simulink model "dc_motor_PI_z"  (R2024a)
settings: Solver=VariableStepAuto  StartTime=0.0  StopTime=5  RelTol=1e-3
undefined symbols (not defined in the file): B, J, Ke, Ki, Kp, Kt, L, R, t_dist, Tl0, Tl1
libraries: slpidlib x1
settings Model: Creator=27165  LastModifiedBy=27165

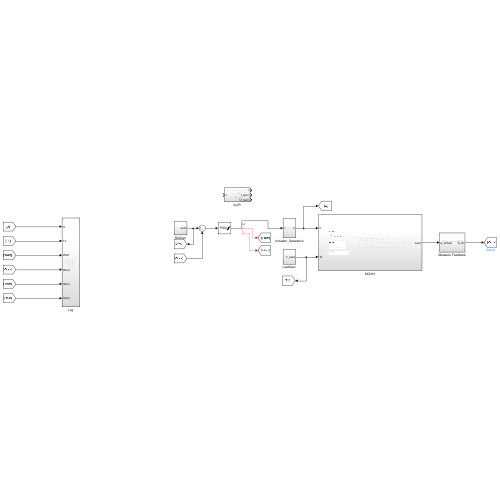
[thumbnail: Simulink's stored preview of the top-level diagram]
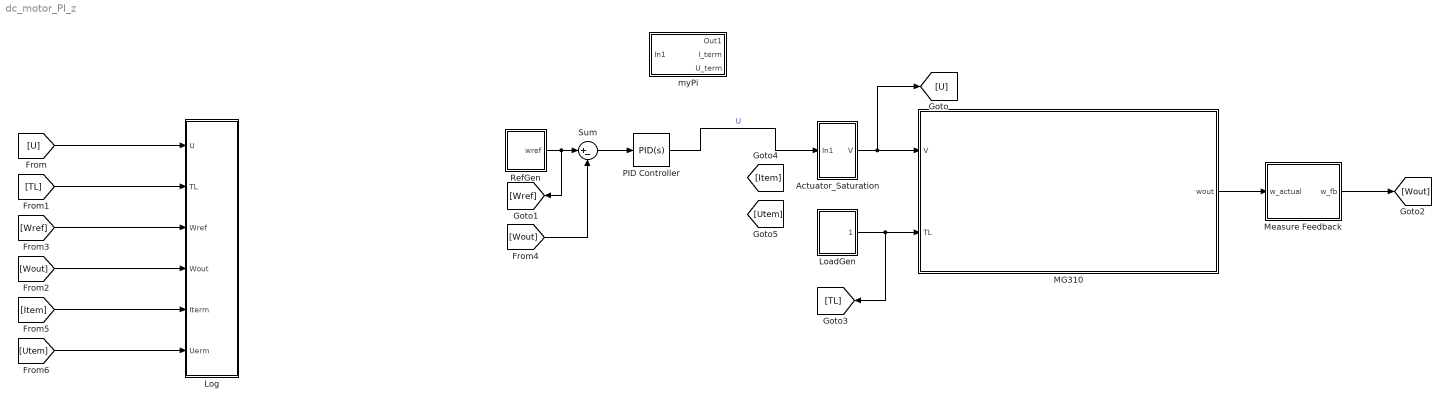
== system dc_motor_PI_z ==
  Actuator_Saturation : Subsystem
  "LoadGen " : Subsystem
  Log : Subsystem
  MG310 : Subsystem
  Measure Feedback : Subsystem
  PID Controller : slpidlib/PID Controller  Controller=PID  Form=Parallel  TimeDomain=Continuous-time  UseExternalTs=off  SampleTime=-1  IntegratorMethod=Forward Euler  FilterMethod=Forward Euler  ControllerParametersSource=internal  P=Kp  I=Ki  UseKiTs=off  D=0  UseExternalDerivativeSource=off  N=100  UseFilter=on  TunerSelectOption=Transfer Function Based (PID Tuner App)  InitialConditionSource=internal  InitialConditionForIntegrator=0  InitialConditionForFilter=0  DifferentiatorICPrevScaledInput=0  ExternalReset=none  TrackingMode=off  Kt=1  LimitOutput=on  SatLimitsSource=internal  UpperSaturationLimit=7.4  LowerSaturationLimit=-7.4  LinearizeAsGain=on  AntiWindupMode=back-calculation  Kb=1000  LimitIntegrator=on  UpperIntegratorSaturationLimit=7.4  LowerIntegratorSaturationLimit=-7.4  POutMin=[]  POutMax=[]  IOutMin=[]  IOutMax=[]  DOutMin=[]  DOutMax=[]  NOutMin=[]  NOutMax=[]  SumOutMin=[]  SumOutMax=[]  SaturationOutMin=[]  SaturationOutMax=[]  PParamMin=[]  PParamMax=[]  IParamMin=[]  IParamMax=[]  DParamMin=[]  DParamMax=[]  NParamMin=[]  NParamMax=[]  KbParamMin=[]  KbParamMax=[]  KtParamMin=[]  KtParamMax=[]  KbOutMin=[]  KbOutMax=[]  KtOutMin=[]  KtOutMax=[]  IntegratorOutMin=[]  IntegratorOutMax=[]  FilterOutMin=[]  FilterOutMax=[]  SumI1OutMin=[]  SumI1OutMax=[]  SumI2OutMin=[]  SumI2OutMax=[]  SumI3OutMin=[]  SumI3OutMax=[]  SumI4OutMin=[]  SumI4OutMax=[]  SumDOutMin=[]  SumDOutMax=[]  DifferentiatorOutMin=[]  DifferentiatorOutMax=[]  FilterDiffOutCoefMin=[]  FilterDiffOutCoefMax=[]  ReciprocalOutMin=[]  ReciprocalOutMax=[]  SumDenOutMin=[]  SumDenOutMax=[]  SumNumOutMin=[]  SumNumOutMax=[]  DivideOutMin=[]  DivideOutMax=[]  UdiffTsProdOutMin=[]  UdiffTsProdOutMax=[]  NTsProdOutMin=[]  NTsProdOutMax=[]  UintegralTsProdOutMin=[]  UintegralTsProdOutMax=[]  UngainTsProdOutMin=[]  UngainTsProdOutMax=[]  ClampingZeroOutDataTypeStr=Inherit: Inherit via back propagation  ClampingZeroOutMin=[]  ClampingZeroOutMax=[]  FilterDenConstantOutDataTypeStr=Inherit: Inherit via back propagation  FilterDenConstantOutMin=[]  FilterDenConstantOutMax=[]  PCopyOutDataTypeStr=Inherit: Inherit via back propagation  PCopyOutMin=[]  PCopyOutMax=[]  NCopyOutDataTypeStr=Inherit: Inherit via back propagation  NCopyOutMin=[]  NCopyOutMax=[]  IntegratorContinuousStateAttributes=''  IntegratorStateMustResolveToSignalObject=off  IntegratorRTWStateStorageClass=Auto  FilterContinuousStateAttributes=''  FilterStateMustResolveToSignalObject=off  FilterRTWStateStorageClass=Auto  ParallelPVariant=InternalParameters  IdealPVariant=Disabled  IVariant=InternalParameters  DVariant=InternalParameters  IntegratorVariant=Continuous  SatVariant=Enabled  AWVariant=BackCalculation  PCopyVariant=Disabled  TRVariant=Disabled  FdbkBlocksVariant=Forward  IdealPFdbkVariant=Disabled  SatFdbkVariant=Disabled  DerivativeFilterVariant=ContFilter  NVariant=InternalParameters  NCopyVariant=Disabled  FilterICVariant=InternalICsFilter  IntegratorICVariant=InternalICs  ExternalResetVariant=Disabled  TRSumVariant=Passthrough  SumFdbkVariant=Disabled  SumVariant=Sum_PID  TsampFilterVariant=InternalTs  TsampNgainVariant=Passthrough  TsampIntegralVariant=Disabled_SignalSpec  ExternalSaturationOutDataTypeStr=Inherit: Same as second input  DerivativeSourceVariant=ErrorSignal
  RefGen : Subsystem
  Sum : Sum  Inputs=|+-
  myPi : Subsystem
  wires:
  Measure Feedback/1(w_fb) -> [Wout]
  [Wout] -> Sum/2
  RefGen/1(wref) -> [Wref], Sum/1
  PID Controller/1 -> Actuator_Saturation/1(In1)  "U"
  Actuator_Saturation/1(V) -> [U], MG310/1(V)
  "LoadGen "/1(T_load) -> [TL], MG310/2(TL)
  MG310/1(wout) -> Measure Feedback/1(w_actual)
  [Wout] -> Log/4(Wout)
  [U] -> Log/1(U)
  [TL] -> Log/2(TL)
  [Wref] -> Log/3(Wref)
  Sum/1 -> PID Controller/1
  ? -> [Item]
  ? -> [Utem]
  [Item] -> Log/5(Iterm)
  [Utem] -> Log/6(Uerm)

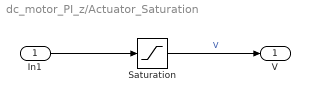
== system dc_motor_PI_z/Actuator_Saturation ==
  In1 : Inport
  Saturation : Saturate  UpperLimit=7.4  LowerLimit=-7.4
  V : Outport
  wires:
  In1/1 -> Saturation/1
  Saturation/1 -> V/1  "V"

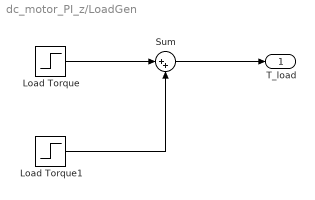
== system dc_motor_PI_z/LoadGen  ==
  Load Torque : Step  Time=t_dist  Before=Tl0  After=Tl1  SampleTime=0
  Load Torque1 : Step  Time=t_dist+2  After=Tl1*-1  SampleTime=0
  Sum : Sum  Inputs=|++
  T_load : Outport
  wires:
  Load Torque/1 -> Sum/1
  Load Torque1/1 -> Sum/2
  Sum/1 -> T_load/1

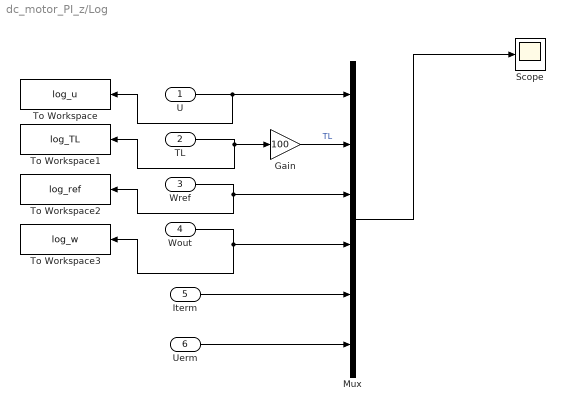
== system dc_motor_PI_z/Log ==
  U : Inport
  TL : Inport  Port=2
  Wref : Inport  Port=3
  Wout : Inport  Port=4
  Iterm : Inport  Port=5
  Uerm : Inport  Port=6
  Gain : Gain  Gain=100
  Mux : Mux  Inputs=6
  Scope : Scope
  To Workspace : ToWorkspace  VariableName=log_u  SaveFormat=Structure With Time  SampleTime=-1
  To Workspace1 : ToWorkspace  VariableName=log_TL  SaveFormat=Structure With Time  SampleTime=-1
  To Workspace2 : ToWorkspace  VariableName=log_ref  SaveFormat=Structure With Time  SampleTime=-1
  To Workspace3 : ToWorkspace  VariableName=log_w  SaveFormat=Structure With Time  SampleTime=-1
  wires:
  Wout/1 -> To Workspace3/1, Mux/4
  U/1 -> To Workspace/1, Mux/1
  TL/1 -> To Workspace1/1, Gain/1
  Wref/1 -> To Workspace2/1, Mux/3
  Gain/1 -> Mux/2  "TL"
  Mux/1 -> Scope/1
  Iterm/1 -> Mux/5
  Uerm/1 -> Mux/6

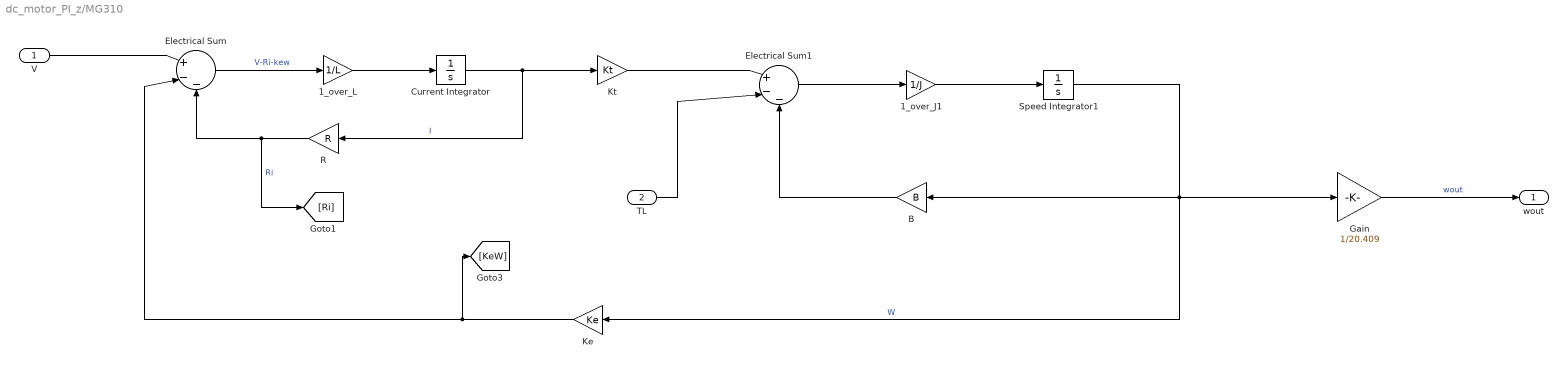
== system dc_motor_PI_z/MG310 ==
  V : Inport
  TL : Inport  Port=2
  1_over_J1 : Gain  Gain=1/J
  1_over_L : Gain  Gain=1/L
  B : Gain  Gain=B
  Current Integrator : Integrator
  Electrical Sum : Sum  Inputs=|+--
  Electrical Sum1 : Sum  Inputs=|+--
  Gain : Gain  Gain=1/20.409
  Ke : Gain  Gain=Ke
  Kt : Gain  Gain=Kt
  R : Gain  Gain=R
  Speed Integrator1 : Integrator
  wout : Outport
  wires:
  R/1 -> [Ri], Electrical Sum/3  "Ri"
  Ke/1 -> [KeW], Electrical Sum/2
  1_over_J1/1 -> Speed Integrator1/1
  Current Integrator/1 -> Kt/1, R/1  "I"
  1_over_L/1 -> Current Integrator/1
  B/1 -> Electrical Sum1/3
  V/1 -> Electrical Sum/1
  Kt/1 -> Electrical Sum1/1
  Speed Integrator1/1 -> Gain/1, Ke/1, B/1  "W"
  TL/1 -> Electrical Sum1/2
  Electrical Sum/1 -> 1_over_L/1  "V-Ri-kew"
  Electrical Sum1/1 -> 1_over_J1/1
  Gain/1 -> wout/1  "wout"

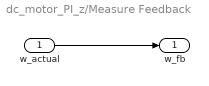
== system dc_motor_PI_z/Measure Feedback ==
  w_actual : Inport
  w_fb : Outport
  wires:
  w_actual/1 -> w_fb/1

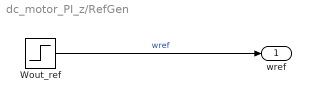
== system dc_motor_PI_z/RefGen ==
  Wout_ref : Step  Time=0.5  After=7  SampleTime=0
  wref : Outport
  wires:
  Wout_ref/1 -> wref/1  "wref"

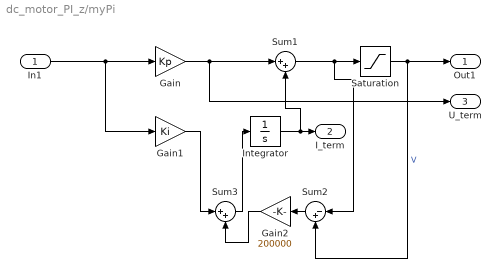
== system dc_motor_PI_z/myPi ==
  In1 : Inport
  Gain : Gain  Gain=Kp
  Gain1 : Gain  Gain=Ki
  Gain2 : Gain  Gain=200000
  Integrator : Integrator
  Saturation : Saturate  UpperLimit=7.4  LowerLimit=0
  Sum1 : Sum  Inputs=|++
  Sum2 : Sum  Inputs=|-+
  Sum3 : Sum  Inputs=|++
  Out1 : Outport
  I_term : Outport  Port=2
  U_term : Outport  Port=3
  wires:
  Gain/1 -> U_term/1, Sum1/1
  Sum1/1 -> Sum2/1, Saturation/1
  In1/1 -> Gain1/1, Gain/1
  Gain1/1 -> Sum3/1
  Saturation/1 -> Sum2/2, Out1/1  "V"
  Sum2/1 -> Gain2/1
  Gain2/1 -> Sum3/2
  Sum3/1 -> Integrator/1
  Integrator/1 -> Sum1/2, I_term/1
